simulink model "assignment2_pruned_2022"  (R2022a)
settings: Solver=FixedStepDiscrete  StartTime=0.0  StopTime=1  FixedStep=0.001  RelTol=1e-3
libraries: dspindex x2, my_neural x2, neural x2, simulink x1, dspsigattribs x1, hdlsllib x1, my_support_func x1
settings Model: DataTypeOverride=Off  Creator=13698  LastModifiedBy=omnipresent
settings OptimizationCC: BlockReduction=off  ConditionallyExecuteInputs=off  DefaultParameterBehavior=Inlined  InheritOutputTypeSmallerThanSingle=on
settings DebuggingCC: AlgebraicLoopMsg=error  SingleTaskRateTransMsg=error  ParameterOverflowMsg=none
settings HardwareCC: ProdBitPerPointer=32  ProdBitPerSizeT=32  ProdBitPerPtrDiffT=32  ProdLargestAtomicFloat=None  ProdIntDivRoundTo=Undefined  ProdEndianess=Unspecified  ProdWordSize=32  ProdHWDeviceType=ASIC/FPGA->ASIC/FPGA  TargetBitPerLong=64  TargetBitPerPointer=64  TargetBitPerSizeT=64  TargetBitPerPtrDiffT=64  TargetLongLongMode=on  TargetIntDivRoundTo=Zero  TargetEndianess=LittleEndian  TargetWordSize=64  TargetHWDeviceType=Custom Processor->MATLAB Host Computer  ProdEqTarget=off
settings ModelReferenceCC: EnableRefExpFcnMdlSchedulingChecks=off
settings RTWCC: Description=Generic Real-Time Target

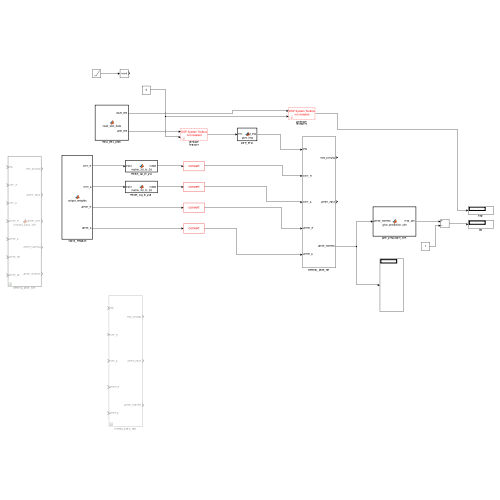
[thumbnail: Simulink's stored preview of the top-level diagram]
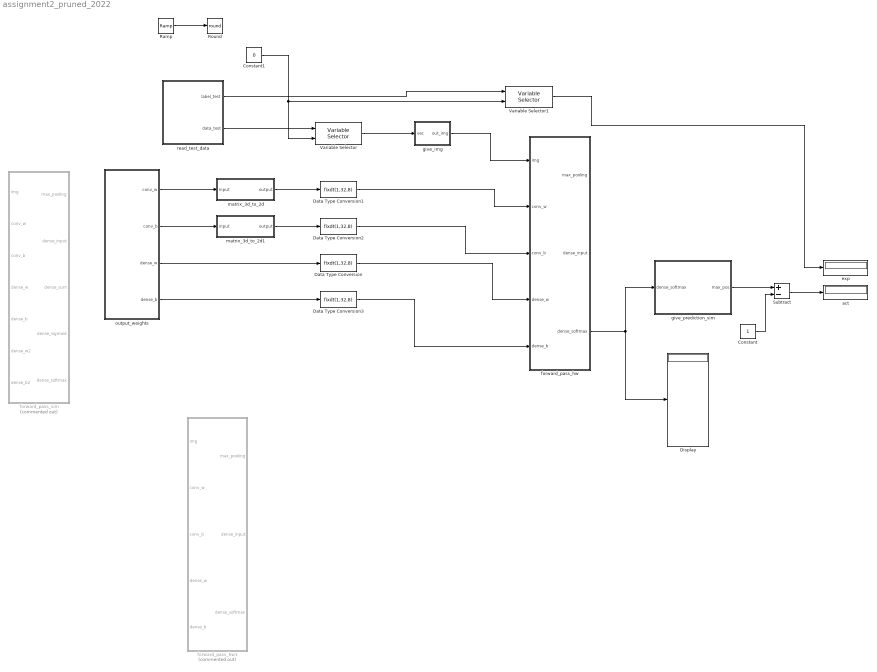
== system assignment2_pruned_2022 ==
  Constant : Constant  OutDataTypeStr=single
  Constant1 : Constant  Value=0
  Data Type Conversion{,1..3} (4 alike) : DataTypeConversion  OutDataTypeStr=fixdt(1,32,8)  SaturateOnIntegerOverflow=off  RndMeth=Floor
  Display : Display
  Ramp : simulink/Sources/Ramp  slope=1  start=0  InitialOutput=0
  Round : Rounding  Operator=round
  Subtract : Sum  Inputs=+-
  Variable Selector : dspindex/Variable Selector  NumInputs=1  rowsOrCols=Rows  IdxMode=Variable  Elements=[1 3]  ZerOneIdxMode=Zero-based  errmode=Generate Error  FillMode=on  FillValues=0
  Variable Selector1 : dspindex/Variable Selector  NumInputs=1  rowsOrCols=Columns  IdxMode=Variable  Elements=[1 3]  ZerOneIdxMode=Zero-based  errmode=Clip Index  FillMode=on  FillValues=0
  act : Display
  exp : Display
  forward_pass_hw : Subsystem
  forward_pass_hw1 : Subsystem  Commented=on
  forward_pass_sim : MATLAB Function  Commented=on  TreatAsAtomicUnit=on
  give_img : MATLAB Function  TreatAsAtomicUnit=on
  give_prediction_sim : MATLAB Function  TreatAsAtomicUnit=on
  matrix_3d_to_2d : MATLAB Function  TreatAsAtomicUnit=on
  matrix_3d_to_2d1 : MATLAB Function  TreatAsAtomicUnit=on
  output_weights : MATLAB Function  TreatAsAtomicUnit=on
  read_test_data : MATLAB Function  TreatAsAtomicUnit=on
  wires:
  Variable Selector/1 -> give_img/1(vec)
  read_test_data/1(label_test) -> Variable Selector1/1
  Variable Selector1/1 -> exp/1
  read_test_data/2(data_test) -> Variable Selector/1
  Subtract/1 -> act/1
  give_prediction_sim/1(max_pos) -> Subtract/1
  Constant/1 -> Subtract/2
  forward_pass_hw/3(dense_softmax) -> Display/1, give_prediction_sim/1(dense_softmax)
  output_weights/3(dense_w) -> Data Type Conversion/1
  output_weights/4(dense_b) -> Data Type Conversion3/1
  Ramp/1 -> Round/1
  Constant1/1 -> Variable Selector1/2, Variable Selector/2
  give_img/1(out_img) -> forward_pass_hw/1(img)
  matrix_3d_to_2d/1(output) -> Data Type Conversion1/1
  matrix_3d_to_2d1/1(output) -> Data Type Conversion2/1
  output_weights/1(conv_w) -> matrix_3d_to_2d/1(input)
  output_weights/2(conv_b) -> matrix_3d_to_2d1/1(input)
  Data Type Conversion/1 -> forward_pass_hw/4(dense_w)
  Data Type Conversion3/1 -> forward_pass_hw/5(dense_b)
  Data Type Conversion1/1 -> forward_pass_hw/2(conv_w)
  Data Type Conversion2/1 -> forward_pass_hw/3(conv_b)

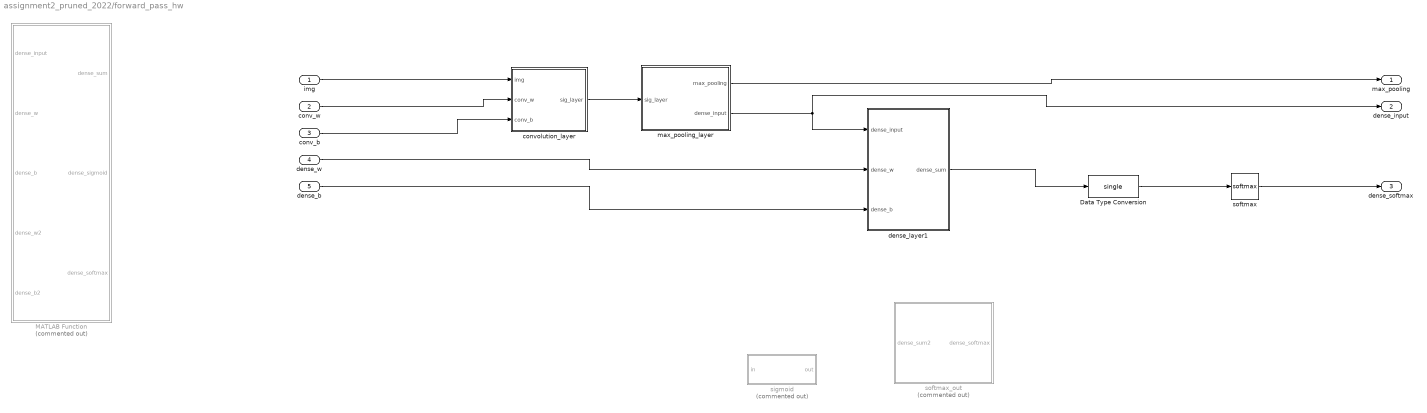
== system assignment2_pruned_2022/forward_pass_hw ==
  img : Inport
  conv_w : Inport  Port=2
  conv_b : Inport  Port=3
  dense_w : Inport  Port=4
  dense_b : Inport  Port=5
  Data Type Conversion : DataTypeConversion  OutDataTypeStr=single  SaturateOnIntegerOverflow=off  RndMeth=Floor
  MATLAB Function : MATLAB Function  Commented=on  TreatAsAtomicUnit=on
  convolution_layer : Subsystem
  dense_layer1 : Subsystem
  max_pooling_layer : MATLAB Function  TreatAsAtomicUnit=on
  sigmoid : Subsystem  Commented=on
  softmax : my_neural/Transfer Functions/softmax
  softmax_out : Subsystem  Commented=on
  max_pooling : Outport
  dense_input : Outport  Port=2
  dense_softmax : Outport  Port=3
  wires:
  convolution_layer/1(sig_layer) -> max_pooling_layer/1(sig_layer)
  max_pooling_layer/2(dense_input) -> dense_layer1/1(dense_input), dense_input/1
  max_pooling_layer/1(max_pooling) -> max_pooling/1
  softmax/1 -> dense_softmax/1
  dense_layer1/1(dense_sum) -> Data Type Conversion/1
  dense_w/1 -> dense_layer1/2(dense_w)
  dense_b/1 -> dense_layer1/3(dense_b)
  conv_w/1 -> convolution_layer/2(conv_w)
  img/1 -> convolution_layer/1(img)
  conv_b/1 -> convolution_layer/3(conv_b)
  Data Type Conversion/1 -> softmax/1

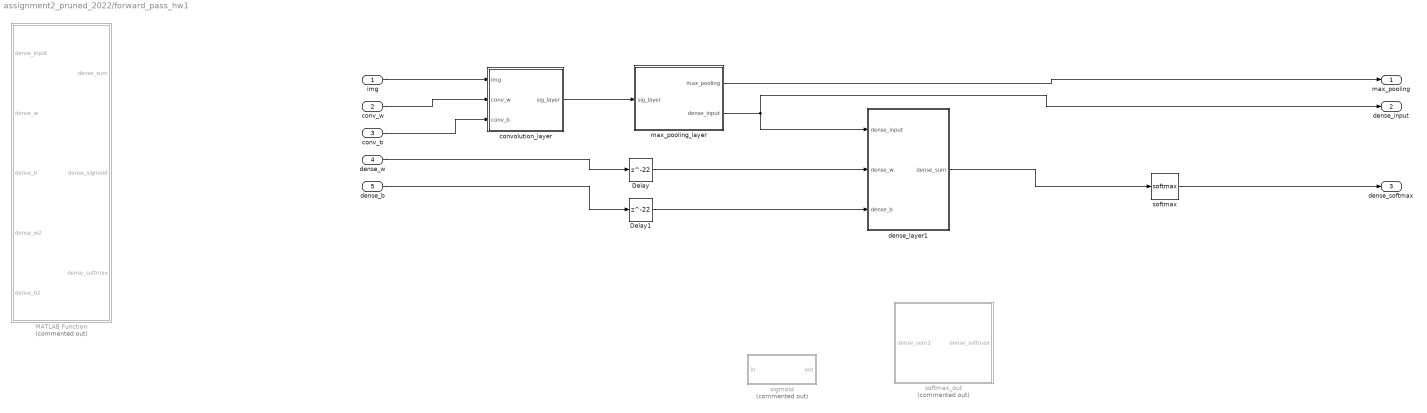
== system assignment2_pruned_2022/forward_pass_hw1 ==
  img : Inport
  conv_w : Inport  Port=2
  conv_b : Inport  Port=3
  dense_w : Inport  Port=4
  dense_b : Inport  Port=5
  Delay : Delay  DelayLength=22
  Delay1 : Delay  DelayLength=22
  MATLAB Function : MATLAB Function  Commented=on  TreatAsAtomicUnit=on
  convolution_layer : Subsystem
  dense_layer1 : Subsystem
  max_pooling_layer : MATLAB Function  TreatAsAtomicUnit=on
  sigmoid : Subsystem  Commented=on
  softmax : neural/Transfer Functions/softmax
  softmax_out : Subsystem  Commented=on
  max_pooling : Outport
  dense_input : Outport  Port=2
  dense_softmax : Outport  Port=3
  wires:
  img/1 -> convolution_layer/1(img)
  conv_w/1 -> convolution_layer/2(conv_w)
  conv_b/1 -> convolution_layer/3(conv_b)
  convolution_layer/1(sig_layer) -> max_pooling_layer/1(sig_layer)
  max_pooling_layer/2(dense_input) -> dense_input/1, dense_layer1/1(dense_input)
  max_pooling_layer/1(max_pooling) -> max_pooling/1
  dense_w/1 -> Delay/1
  dense_b/1 -> Delay1/1
  softmax/1 -> dense_softmax/1
  dense_layer1/1(dense_sum) -> softmax/1
  Delay/1 -> dense_layer1/2(dense_w)
  Delay1/1 -> dense_layer1/3(dense_b)

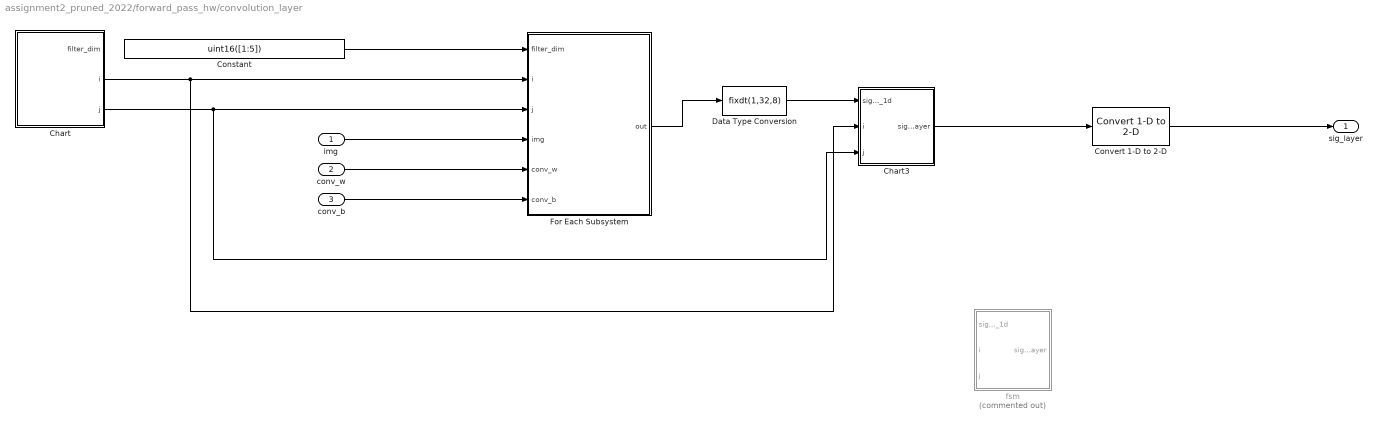
== system assignment2_pruned_2022/forward_pass_hw/convolution_layer ==
  img : Inport
  conv_w : Inport  Port=2
  conv_b : Inport  Port=3
  Chart : Stateflow chart  TreatAsAtomicUnit=on
  Chart3 : Stateflow chart  TreatAsAtomicUnit=on
  Constant : Constant  Value=uint16([1:5])  SampleTime=-1
  Convert 1-D to 2-D : dspsigattribs/Convert 1-D to 2-D  M=5  N=784  frameBasedOut=off
  Data Type Conversion : DataTypeConversion  OutDataTypeStr=fixdt(1,32,8)  SaturateOnIntegerOverflow=off  RndMeth=Floor
  For Each Subsystem : Subsystem  TreatAsAtomicUnit=on
  fsm : Stateflow chart  Commented=on  TreatAsAtomicUnit=on
  sig_layer : Outport
  wires:
  img/1 -> For Each Subsystem/4(img)
  conv_w/1 -> For Each Subsystem/5(conv_w)
  conv_b/1 -> For Each Subsystem/6(conv_b)
  For Each Subsystem/1(out) -> Data Type Conversion/1
  Data Type Conversion/1 -> Chart3/1(sig_layer_1d)
  Chart3/1(sig_layer) -> Convert 1-D to 2-D/1
  Convert 1-D to 2-D/1 -> sig_layer/1
  Chart/3(j) -> Chart3/3(j), For Each Subsystem/3(j)
  Chart/2(i) -> Chart3/2(i), For Each Subsystem/2(i)
  Constant/1 -> For Each Subsystem/1(filter_dim)

== system assignment2_pruned_2022/forward_pass_hw/dense_layer1 ==
  dense_input : Inport
  dense_w : Inport  Port=2
  dense_b : Inport  Port=3
  For Each Subsystem : Subsystem  TreatAsAtomicUnit=on
  dense_sum : Outport
  wires:
  dense_input/1 -> For Each Subsystem/1(dense_input)
  dense_w/1 -> For Each Subsystem/2(dense_w)
  dense_b/1 -> For Each Subsystem/3(dense_b)
  For Each Subsystem/1(dense_sum) -> dense_sum/1

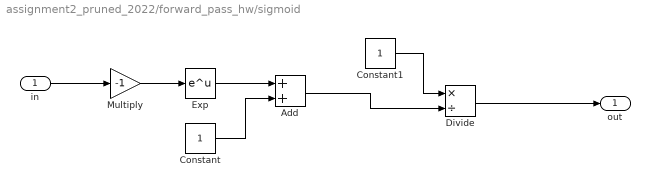
== system assignment2_pruned_2022/forward_pass_hw/sigmoid ==
  in : Inport
  Add : Sum
  Constant : Constant
  Constant1 : Constant
  Divide : Product  Inputs=*/
  Exp : Math
  Multiply : Gain  Gain=-1
  out : Outport
  wires:
  in/1 -> Multiply/1
  Multiply/1 -> Exp/1
  Exp/1 -> Add/1
  Constant/1 -> Add/2
  Divide/1 -> out/1
  Add/1 -> Divide/2
  Constant1/1 -> Divide/1

== system assignment2_pruned_2022/forward_pass_hw/softmax_out ==
  dense_sum2 : Inport
  Exp : Math
  For Each Subsystem : Subsystem  TreatAsAtomicUnit=on
  Sum of Elements : Sum  Inputs=+
  dense_softmax : Outport
  wires:
  dense_sum2/1 -> Exp/1
  Exp/1 -> For Each Subsystem/2(exp_dense_sum2), Sum of Elements/1
  For Each Subsystem/1(dense_softmax) -> dense_softmax/1
  Sum of Elements/1 -> For Each Subsystem/1(den)

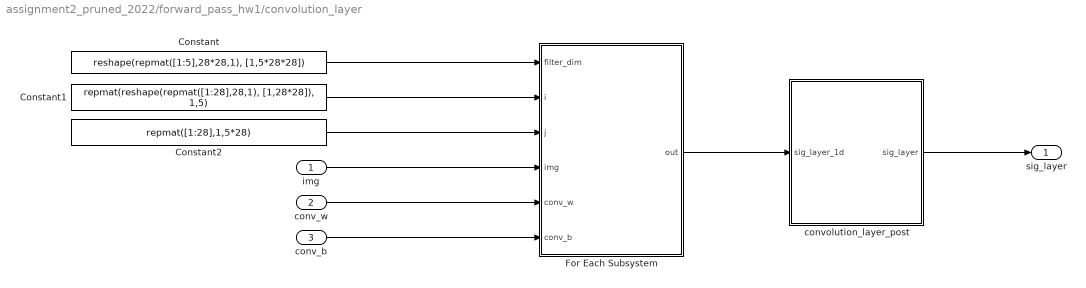
== system assignment2_pruned_2022/forward_pass_hw1/convolution_layer ==
  img : Inport
  conv_w : Inport  Port=2
  conv_b : Inport  Port=3
  Constant : Constant  Value=reshape(repmat([1:5],28*28,1), [1,5*28*28])  OutDataTypeStr=single  SampleTime=-1
  Constant1 : Constant  Value=repmat(reshape(repmat([1:28],28,1), [1,28*28]), 1,5)  OutDataTypeStr=single  SampleTime=-1
  Constant2 : Constant  Value=repmat([1:28],1,5*28)  OutDataTypeStr=single  SampleTime=-1
  For Each Subsystem : Subsystem  TreatAsAtomicUnit=on
  convolution_layer_post : MATLAB Function  TreatAsAtomicUnit=on
  sig_layer : Outport
  wires:
  img/1 -> For Each Subsystem/4(img)
  conv_w/1 -> For Each Subsystem/5(conv_w)
  conv_b/1 -> For Each Subsystem/6(conv_b)
  Constant/1 -> For Each Subsystem/1(filter_dim)
  Constant1/1 -> For Each Subsystem/2(i)
  Constant2/1 -> For Each Subsystem/3(j)
  For Each Subsystem/1(out) -> convolution_layer_post/1(sig_layer_1d)
  convolution_layer_post/1(sig_layer) -> sig_layer/1

== system assignment2_pruned_2022/forward_pass_hw1/dense_layer1 ==
  dense_input : Inport
  dense_w : Inport  Port=2
  dense_b : Inport  Port=3
  For Each Subsystem : Subsystem  TreatAsAtomicUnit=on
  dense_sum : Outport
  wires:
  dense_input/1 -> For Each Subsystem/1(dense_input)
  dense_w/1 -> For Each Subsystem/2(dense_w)
  dense_b/1 -> For Each Subsystem/3(dense_b)
  For Each Subsystem/1(dense_sum) -> dense_sum/1

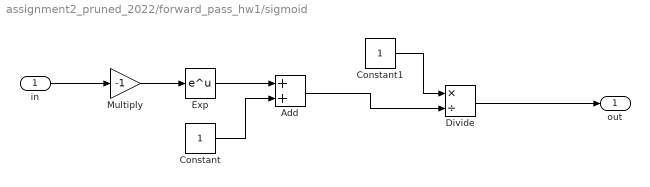
== system assignment2_pruned_2022/forward_pass_hw1/sigmoid ==
  in : Inport
  Add : Sum
  Constant : Constant
  Constant1 : Constant
  Divide : Product  Inputs=*/
  Exp : Math
  Multiply : Gain  Gain=-1
  out : Outport
  wires:
  in/1 -> Multiply/1
  Multiply/1 -> Exp/1
  Exp/1 -> Add/1
  Constant/1 -> Add/2
  Divide/1 -> out/1
  Add/1 -> Divide/2
  Constant1/1 -> Divide/1

== system assignment2_pruned_2022/forward_pass_hw1/softmax_out ==
  dense_sum2 : Inport
  Exp : Math
  For Each Subsystem : Subsystem  TreatAsAtomicUnit=on
  Sum of Elements : Sum  Inputs=+
  dense_softmax : Outport
  wires:
  dense_sum2/1 -> Exp/1
  Exp/1 -> For Each Subsystem/2(exp_dense_sum2), Sum of Elements/1
  For Each Subsystem/1(dense_softmax) -> dense_softmax/1
  Sum of Elements/1 -> For Each Subsystem/1(den)

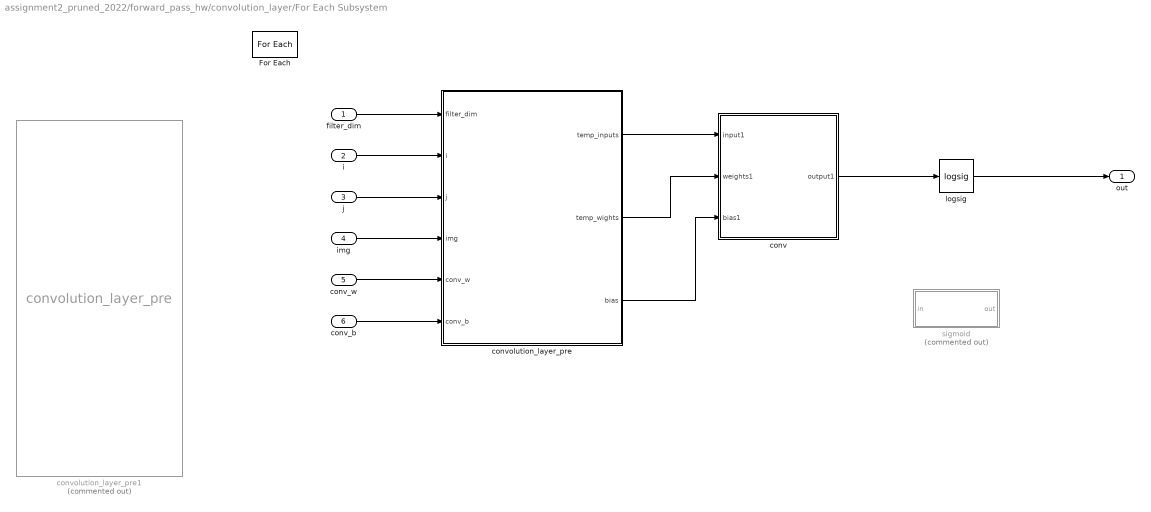
== system assignment2_pruned_2022/forward_pass_hw/convolution_layer/For Each Subsystem ==
  filter_dim : Inport  Partition=on  PartitionDimension=1  PartitionWidth=1  PartitionOffset=0
  i : Inport  Port=2
  j : Inport  Port=3
  img : Inport  Port=4
  conv_w : Inport  Port=5
  conv_b : Inport  Port=6
  For Each : ForEach  DisableCoverage=on
  conv : Subsystem
  convolution_layer_pre : MATLAB Function  TreatAsAtomicUnit=on
  convolution_layer_pre1 : my_support_func/convolution_layer_pre  Commented=on  SampleTime=-1
  logsig : my_neural/Transfer Functions/logsig
  sigmoid : Subsystem  Commented=on
  out : Outport  ConcatenationDimension=1
  wires:
  logsig/1 -> out/1
  conv/1(output1) -> logsig/1
  filter_dim/1 -> convolution_layer_pre/1(filter_dim)
  i/1 -> convolution_layer_pre/2(i)
  j/1 -> convolution_layer_pre/3(j)
  img/1 -> convolution_layer_pre/4(img)
  conv_w/1 -> convolution_layer_pre/5(conv_w)
  conv_b/1 -> convolution_layer_pre/6(conv_b)
  convolution_layer_pre/1(temp_inputs) -> conv/1(input1)
  convolution_layer_pre/2(temp_wights) -> conv/2(weights1)
  convolution_layer_pre/3(bias) -> conv/3(bias1)

== system assignment2_pruned_2022/forward_pass_hw/dense_layer1/For Each Subsystem ==
  dense_input : Inport
  dense_w : Inport  Port=2  Partition=on  PartitionDimension=2  PartitionWidth=1  PartitionOffset=0
  dense_b : Inport  Port=3  Partition=on  PartitionDimension=2  PartitionWidth=1  PartitionOffset=0
  For Each : ForEach  DisableCoverage=on
  conv : Subsystem
  dense_sum : Outport  ConcatenationDimension=1
  wires:
  dense_input/1 -> conv/1(input)
  dense_b/1 -> conv/3(bias)
  conv/1(output) -> dense_sum/1
  dense_w/1 -> conv/2(weights)

== system assignment2_pruned_2022/forward_pass_hw/softmax_out/For Each Subsystem ==
  den : Inport
  exp_dense_sum2 : Inport  Port=2  Partition=on  PartitionDimension=1  PartitionWidth=1  PartitionOffset=0
  Divide : Product  Inputs=*/
  For Each : ForEach  DisableCoverage=on
  dense_softmax : Outport  ConcatenationDimension=1
  wires:
  Divide/1 -> dense_softmax/1
  exp_dense_sum2/1 -> Divide/1
  den/1 -> Divide/2

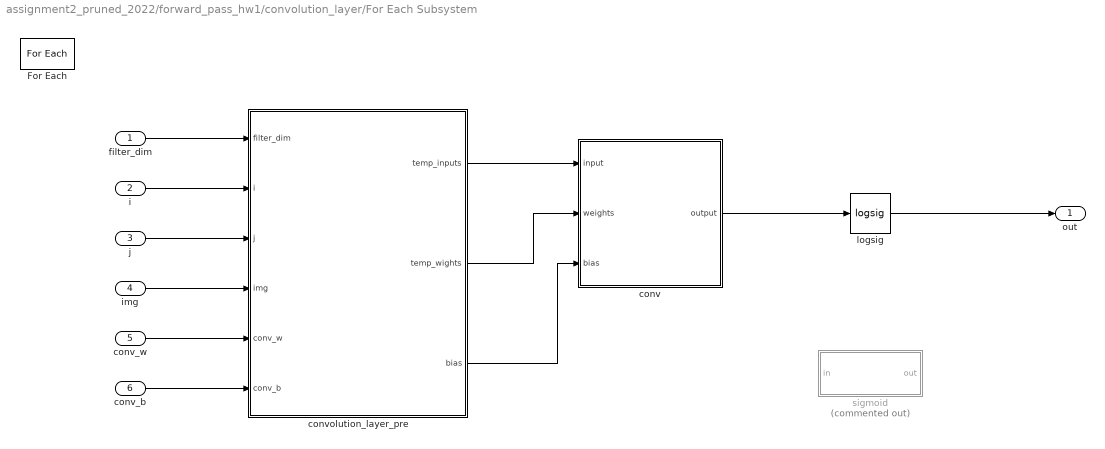
== system assignment2_pruned_2022/forward_pass_hw1/convolution_layer/For Each Subsystem ==
  filter_dim : Inport  Partition=on  PartitionDimension=1  PartitionWidth=1  PartitionOffset=0
  i : Inport  Port=2  Partition=on  PartitionDimension=1  PartitionWidth=1  PartitionOffset=0
  j : Inport  Port=3  Partition=on  PartitionDimension=1  PartitionWidth=1  PartitionOffset=0
  img : Inport  Port=4
  conv_w : Inport  Port=5
  conv_b : Inport  Port=6
  For Each : ForEach  DisableCoverage=on
  conv : Subsystem
  convolution_layer_pre : MATLAB Function  TreatAsAtomicUnit=on
  logsig : neural/Transfer Functions/logsig
  sigmoid : Subsystem  Commented=on
  out : Outport  ConcatenationDimension=1
  wires:
  convolution_layer_pre/1(temp_inputs) -> conv/1(input)
  convolution_layer_pre/2(temp_wights) -> conv/2(weights)
  convolution_layer_pre/3(bias) -> conv/3(bias)
  filter_dim/1 -> convolution_layer_pre/1(filter_dim)
  i/1 -> convolution_layer_pre/2(i)
  j/1 -> convolution_layer_pre/3(j)
  img/1 -> convolution_layer_pre/4(img)
  conv_w/1 -> convolution_layer_pre/5(conv_w)
  conv_b/1 -> convolution_layer_pre/6(conv_b)
  conv/1(output) -> logsig/1
  logsig/1 -> out/1

== system assignment2_pruned_2022/forward_pass_hw1/dense_layer1/For Each Subsystem ==
  dense_input : Inport
  dense_w : Inport  Port=2  Partition=on  PartitionDimension=2  PartitionWidth=1  PartitionOffset=0
  dense_b : Inport  Port=3  Partition=on  PartitionDimension=2  PartitionWidth=1  PartitionOffset=0
  For Each : ForEach  DisableCoverage=on
  conv : Subsystem
  dense_sum : Outport  ConcatenationDimension=1
  wires:
  dense_input/1 -> conv/1(input)
  dense_b/1 -> conv/3(bias)
  conv/1(output) -> dense_sum/1
  dense_w/1 -> conv/2(weights)

== system assignment2_pruned_2022/forward_pass_hw1/softmax_out/For Each Subsystem ==
  den : Inport
  exp_dense_sum2 : Inport  Port=2  Partition=on  PartitionDimension=1  PartitionWidth=1  PartitionOffset=0
  Divide : Product  Inputs=*/
  For Each : ForEach  DisableCoverage=on
  dense_softmax : Outport  ConcatenationDimension=1
  wires:
  Divide/1 -> dense_softmax/1
  exp_dense_sum2/1 -> Divide/1
  den/1 -> Divide/2

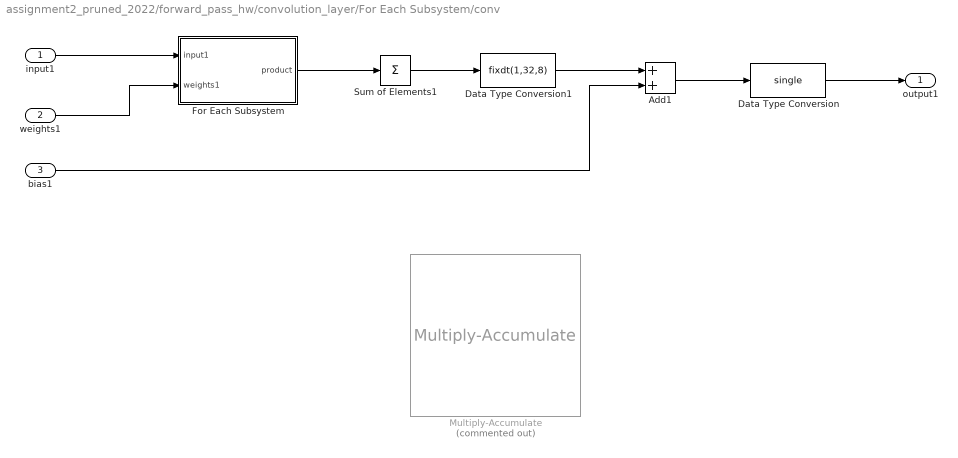
== system assignment2_pruned_2022/forward_pass_hw/convolution_layer/For Each Subsystem/conv ==
  input1 : Inport
  weights1 : Inport  Port=2
  bias1 : Inport  Port=3
  Add1 : Sum
  Data Type Conversion : DataTypeConversion  OutDataTypeStr=single  SaturateOnIntegerOverflow=off  RndMeth=Floor
  Data Type Conversion1 : DataTypeConversion  OutDataTypeStr=fixdt(1,32,8)  SaturateOnIntegerOverflow=off  RndMeth=Floor
  For Each Subsystem : Subsystem  TreatAsAtomicUnit=on
  Multiply-Accumulate : hdlsllib/HDL Operations/Multiply-Accumulate  Commented=on  opMode=Vector  initValueSetting=Input port  initValue=0  initValueSetting2=Dialog  initValue2=0  initValueSetting3=Dialog  initValue3=0  num_samples=2  RndMeth2=Floor  RndMeth3=Floor  OutDataTypeStr=fixdt(1,32,8)  datatype2=Inherit: Inherit via back propagation  datatype3=Inherit: Inherit via back propagation  validOut=on  endInandOut=on  startOut=on  countOut=on  dim=-1  DoSatur=off  parallel=off
  Sum of Elements1 : Sum  Inputs=+
  output1 : Outport
  wires:
  Sum of Elements1/1 -> Data Type Conversion1/1
  bias1/1 -> Add1/2
  Add1/1 -> Data Type Conversion/1
  input1/1 -> For Each Subsystem/1(input1)
  weights1/1 -> For Each Subsystem/2(weights1)
  For Each Subsystem/1(product) -> Sum of Elements1/1
  Data Type Conversion/1 -> output1/1
  Data Type Conversion1/1 -> Add1/1

== system assignment2_pruned_2022/forward_pass_hw/convolution_layer/For Each Subsystem/sigmoid ==
  in : Inport
  Add : Sum
  Constant : Constant
  Constant1 : Constant
  Divide : Product  Inputs=*/
  Exp : Math
  Multiply : Gain  Gain=-1
  out : Outport
  wires:
  in/1 -> Multiply/1
  Multiply/1 -> Exp/1
  Exp/1 -> Add/1
  Constant/1 -> Add/2
  Divide/1 -> out/1
  Add/1 -> Divide/2
  Constant1/1 -> Divide/1

== system assignment2_pruned_2022/forward_pass_hw/dense_layer1/For Each Subsystem/conv ==
  input : Inport
  weights : Inport  Port=2
  bias : Inport  Port=3
  Add : Sum  OutDataTypeStr=Inherit: Inherit via back propagation
  Data Type Conversion : DataTypeConversion  OutDataTypeStr=fixdt(1,32,8)  SaturateOnIntegerOverflow=off  RndMeth=Floor
  For Each Subsystem : Subsystem  TreatAsAtomicUnit=on
  Sum of Elements : Sum  Inputs=+
  output : Outport
  wires:
  Add/1 -> output/1
  Sum of Elements/1 -> Data Type Conversion/1
  bias/1 -> Add/2
  For Each Subsystem/1(product) -> Sum of Elements/1
  input/1 -> For Each Subsystem/1(input1)
  weights/1 -> For Each Subsystem/2(weights1)
  Data Type Conversion/1 -> Add/1

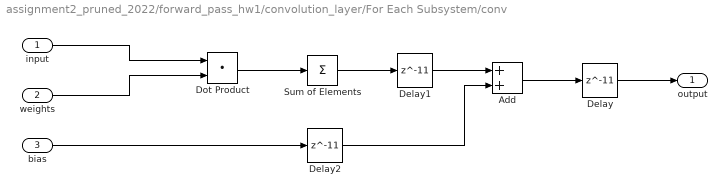
== system assignment2_pruned_2022/forward_pass_hw1/convolution_layer/For Each Subsystem/conv ==
  input : Inport
  weights : Inport  Port=2
  bias : Inport  Port=3
  Add : Sum
  Delay : Delay  DelayLength=11
  Delay1 : Delay  DelayLength=11
  Delay2 : Delay  DelayLength=11
  Dot Product : DotProduct  OutDataTypeStr=Inherit: Inherit via internal rule
  Sum of Elements : Sum  Inputs=+
  output : Outport
  wires:
  input/1 -> Dot Product/1
  weights/1 -> Dot Product/2
  Dot Product/1 -> Sum of Elements/1
  Sum of Elements/1 -> Delay1/1
  bias/1 -> Delay2/1
  Delay/1 -> output/1
  Delay1/1 -> Add/1
  Delay2/1 -> Add/2
  Add/1 -> Delay/1

== system assignment2_pruned_2022/forward_pass_hw1/convolution_layer/For Each Subsystem/sigmoid ==
  in : Inport
  Add : Sum
  Constant : Constant
  Constant1 : Constant
  Divide : Product  Inputs=*/
  Exp : Math
  Multiply : Gain  Gain=-1
  out : Outport
  wires:
  in/1 -> Multiply/1
  Multiply/1 -> Exp/1
  Exp/1 -> Add/1
  Constant/1 -> Add/2
  Divide/1 -> out/1
  Add/1 -> Divide/2
  Constant1/1 -> Divide/1

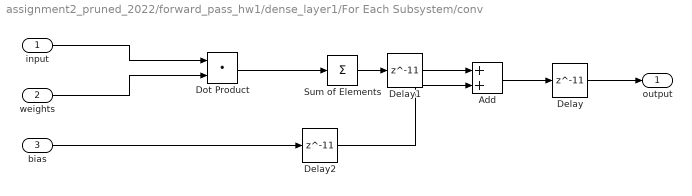
== system assignment2_pruned_2022/forward_pass_hw1/dense_layer1/For Each Subsystem/conv ==
  input : Inport
  weights : Inport  Port=2
  bias : Inport  Port=3
  Add : Sum  OutDataTypeStr=single
  Delay : Delay  DelayLength=11
  Delay1 : Delay  DelayLength=11
  Delay2 : Delay  DelayLength=11
  Dot Product : DotProduct  OutDataTypeStr=Inherit: Inherit via internal rule
  Sum of Elements : Sum  Inputs=+
  output : Outport
  wires:
  input/1 -> Dot Product/1
  weights/1 -> Dot Product/2
  Dot Product/1 -> Sum of Elements/1
  Sum of Elements/1 -> Delay1/1
  Add/1 -> Delay/1
  bias/1 -> Delay2/1
  Delay/1 -> output/1
  Delay1/1 -> Add/1
  Delay2/1 -> Add/2

== system assignment2_pruned_2022/forward_pass_hw/convolution_layer/For Each Subsystem/conv/For Each Subsystem ==
  input1 : Inport  Partition=on  PartitionDimension=2  PartitionWidth=1  PartitionOffset=0
  weights1 : Inport  Port=2  Partition=on  PartitionDimension=2  PartitionWidth=1  PartitionOffset=0
  For Each : ForEach  DisableCoverage=on
  Product : Product
  product : Outport  ConcatenationDimension=1
  wires:
  input1/1 -> Product/1
  weights1/1 -> Product/2
  Product/1 -> product/1

== system assignment2_pruned_2022/forward_pass_hw/dense_layer1/For Each Subsystem/conv/For Each Subsystem ==
  input1 : Inport  Partition=on  PartitionDimension=2  PartitionWidth=1  PartitionOffset=0
  weights1 : Inport  Port=2  Partition=on  PartitionDimension=1  PartitionWidth=1  PartitionOffset=0
  For Each : ForEach  DisableCoverage=on
  Product : Product
  product : Outport  ConcatenationDimension=1
  wires:
  input1/1 -> Product/1
  weights1/1 -> Product/2
  Product/1 -> product/1

== matlab function assignment2_pruned_2022/read_test_data ==
  data: label_test output; data_test output
function [label_test, data_test] = read_test_data()
    data = load('test_set.mat');
    label_test = data.label_test;
    data_test = data.data_test;
end

== matlab function assignment2_pruned_2022/output_weights ==
  data: conv_w output; conv_b output; dense_w output; dense_b output
function [conv_w, conv_b, dense_w, dense_b] = output_weights
    data = load('weights_pruned.mat');
    conv_w = (data.conv_w);
    conv_b = (data.conv_b);
    dense_w = (data.dense_w);
    dense_b = (data.dense_b);
    end

== matlab function assignment2_pruned_2022/give_img ==
  data: vec input; out_img output
function out_img = give_img(vec)
    img = zeros(35,32,'uint8');
    k=1;
    for i=1:35
        for j=1:32
            if (i < 6|| j < 3 || i > 33 || j > 30)
                img(i,j) = 0;
            else
                img(i,j) = vec(k);
                k = k + 1;
            end
        end
    end

    out_img = reshape(transpose(img), [1, length(img(1,:))*length(img)]);
end

== matlab function assignment2_pruned_2022/forward_pass_hw/convolution_layer/For Each Subsystem/convolution_layer_pre ==
  settings: fimath=fimath('RoundingMethod', 'Floor','OverflowAction', 'Wrap','ProductMode', 'FullPrecision', 'SumMode', 'FullPrecision')
  data: filter_dim input; temp_inputs output; i input; j input; img input; conv_w input; conv_b input; temp_wights output; bias output
function [temp_inputs, temp_wights, bias] = convolution_layer_pre(filter_dim, i, j, img, conv_w, conv_b)
    
    % temp_img = reshape(transpose(img), [1, length(img(1,:))*length(img)]);
    
    temp_wights = fi(zeros(1,7*7), 1, 32, 8);
    temp_inputs = fi(zeros(1,7*7), 1, 32, 8);
    i = single(i);
    j = single(j);
    for k=1:7
        for l=1:7
            temp_wights((k-1)*7 + l) = single(img((i + k + 1 - 1 - 1)*32 + j + l - 2 - 1));
            temp_inputs((k-1)*7 + l) = conv_w(filter_dim, (k-1)*7 + l);
        end
    end
    bias = conv_b(filter_dim, (i-1)*28+j);
    
    % temp_wights = zeros(1,7*7, "single");
    % temp_inputs = zeros(1,7*7, "single");
    % for k=1:7
    %     for l=1:7
    %         temp_wights((k-1)*7 + l) = cast(img((i + k + 1 - 1 - 1)*32 + j + l - 2 - 1), 'double');
    %         temp_inputs((k-1)*7 + l) = conv_w(filter_dim, k, l);
    %     end
    % end
    % bias = conv_b(filter_dim, i, j);
end

== matlab function assignment2_pruned_2022/forward_pass_sim ==
  data: img input; max_pooling output; conv_w input; conv_b input; dense_w input; dense_b input; dense_w2 input; dense_b2 input; dense_input output; dense_sum output; dense_sigmoid output; dense_softmax output
function [max_pooling, dense_input, dense_sum, dense_sigmoid, dense_softmax] = forward_pass_sim(img, conv_w, conv_b, dense_w, dense_b, dense_w2, dense_b2)
    max_pooling = zeros(5,28,28);
    dense_input = zeros(1,980);
    dense_sum = zeros(1,120);
    dense_sigmoid = zeros(1,120);
    dense_softmax = zeros(1,10);
    
    conv_layer = zeros(5,28,28);
    sig_layer = zeros(5,28,28);
    max_layer = zeros(5,14,14);
    dense_sum2 = zeros(1,10);
    
    temp_img = reshape(transpose(img), [1, length(img(1,:))*length(img)]);
    
    % Convolution Operation + Sigmoid Activation
    for filter_dim=1:5
        for i=1:28
            for j=1:28
                temp_wights = zeros(1,7*7);
                temp_inputs = zeros(1,7*7);
                for k=1:7
                    for l=1:7
                        temp_wights((k-1)*7 + l) = cast(temp_img((i + k + 1 - 1 - 1)*32 + j + l - 2 - 1), 'double');
                        temp_inputs((k-1)*7 + l) = conv_w(filter_dim, k, l);
                    end
                end
                conv_layer(filter_dim, i, j) = convolusion(temp_inputs, temp_wights, conv_b(filter_dim, i, j));
            end
        end
    end
    sig_layer = 1 ./ (1 + exp(-1 .* conv_layer));
    
    % MAX Pooling (max_pooling, max_layer)
    for filter_dim=1:5
        for i=1:2:28
            for j=1:2:28
                matrix = sig_layer(filter_dim,i:i+1,j:j+1);
                [M,I] = max(matrix);
                [M2,I2] = max(M);
                I = [I(I2) I2];
                max_pooling(filter_dim, I(1), I(2)) = 1;
                max_layer(filter_dim, (i+1)/2, (j+1)/2) = M2;
            end
        end
    end
    for i=1:5
        for j=1:14
            dense_input((i-1)*14*14 + (j-1)*14 + 1 : (i-1)*14*14 + (j-1)*14 + 14) = reshape(max_layer(i,j,:), [1 14]);
        end
    end
    
    % Dense Layer
    for i=1:120
        dense_sum(i) = convolusion(transpose(dense_w(:,i)), dense_input, dense_b(i));
    end
    dense_sigmoid = 1 ./ (1 + exp(-1 .* dense_sum));
    
    % Dense Layer 2
    for i=1:10
        dense_sum2(i) = convolusion(transpose(dense_w2(:,i)), dense_sigmoid, dense_b2(i));
    end
    
    % Softmax Output
    dense_softmax_new = exp(dense_sum2);
    for i=1:10
        dense_softmax(i) = dense_softmax_new(i) / sum(dense_softmax_new);
    end
end

== matlab function assignment2_pruned_2022/forward_pass_hw/MATLAB Function ==
  settings: fimath=fimath('RoundingMethod', 'Floor','OverflowAction', 'Wrap','ProductMode', 'FullPrecision', 'SumMode', 'FullPrecision')
  data: dense_input input; dense_w input; dense_b input; dense_w2 input; dense_b2 input; dense_sum output; dense_sigmoid output; dense_softmax output
function [dense_sum, dense_sigmoid, dense_softmax] = temp(dense_input, dense_w, dense_b, dense_w2, dense_b2)
max_pooling = zeros(5,28,28);
dense_sum = zeros(1,120);
dense_sigmoid = zeros(1,120);
dense_softmax = zeros(1,10);

conv_layer = zeros(5,28,28);
max_layer = zeros(5,14,14);
dense_sum2 = zeros(1,10);

% Dense Layer
for i=1:120
    dense_sum(i) = convolusion(transpose(dense_w(:,i)), dense_input, dense_b(i));
end
dense_sigmoid = 1 ./ (1 + exp(-1 .* dense_sum));

% Dense Layer 2
for i=1:10
    dense_sum2(i) = convolusion(transpose(dense_w2(:,i)), dense_sigmoid, dense_b2(i));
end

% Softmax Output
dense_softmax_new = exp(dense_sum2);
for i=1:10
    dense_softmax(i) = dense_softmax_new(i) / sum(dense_softmax_new);
end

== matlab function assignment2_pruned_2022/forward_pass_hw/max_pooling_layer ==
  settings: fimath=fimath('RoundingMethod', 'Floor','OverflowAction', 'Wrap','ProductMode', 'FullPrecision', 'SumMode', 'FullPrecision')
  data: sig_layer input; max_pooling output; dense_input output
function [max_pooling, dense_input] = max_pooling_layer(sig_layer)

    max_pooling = fi(zeros(5,28*28), 1, 32, 8);
    max_layer = fi(zeros(5,14*14), 1, 32, 8);
    dense_input = fi(zeros(1,980), 1, 32, 8);
    
    % MAX Pooling (max_pooling, max_layer)
    for filter_dim=uint32(1:5)
        for i=uint32(1:2:28)
            for j=uint32(1:2:28)
                matrix = [sig_layer(filter_dim, (i-1)*28+j), sig_layer(filter_dim, (i-1)*28+j+1), sig_layer(filter_dim, (i)*28+j), sig_layer(filter_dim, (i)*28+j+1)];
                M = max(matrix);
                if (M == matrix(1))
                    I = single(1);
                elseif (M == matrix(2))
                    I = single(2);
                elseif (M == matrix(3))
                    I = single(3);
                else
                    I = single(4);
                end
                max_i = uint32(single(i) + ceil(I/2) - 1);
                max_j = uint32(single(j) + 2-mod(I,2) - 1);
                max_pooling(filter_dim, (max_i-1)*28+max_j) = 1;
                max_layer(filter_dim, ((i+1)/2-1)*14+(j+1)/2) = M;
            end
        end
    end
    for i=uint32(1:5)
        dense_input((i-1)*14*14 + 1 : (i-1)*14*14 + 14*14) = reshape(max_layer(i,:), [1 14*14]);
    end
    
    % pooling = zeros(5,28,28, "single");
    % max_layer = zeros(5,14,14, "single");
    % dense_input = zeros(1,980, "single");
    % 
    % % MAX Pooling (max_pooling, max_layer)
    % for filter_dim=1:5
    %     for i=1:2:28
    %         for j=1:2:28
    %             matrix = sig_layer(filter_dim,i:i+1,j:j+1);
    %             [M,I] = max(matrix);
    %             [M2,I2] = max(M);
    %             I = [I(I2) I2];
    %             max_pooling(filter_dim, I(1), I(2)) = 1;
    %             max_layer(filter_dim, (i+1)/2, (j+1)/2) = M2;
    %         end
    %     end
    % end
    % for i=1:5
    %     for j=1:14
    %         dense_input((i-1)*14*14 + (j-1)*14 + 1 : (i-1)*14*14 + (j-1)*14 + 14) = reshape(max_layer(i,j,:), [1 14]);
    %     end
    % end
end

== matlab function assignment2_pruned_2022/give_prediction_sim ==
  data: dense_softmax input; max_pos output
function max_pos = give_prediction_sim(dense_softmax)
    [~,max_pos] = max(dense_softmax);
end

== matlab function assignment2_pruned_2022/matrix_3d_to_2d ==
  data: input input; output output
function output = matrix_3d_to_2d(input)
    matrix_size = size(input);
    output = zeros([matrix_size(1), matrix_size(2) * matrix_size(3)], 'single');
    for i=1:matrix_size(1)
        for j=1:matrix_size(2)
            output(i, (j-1)*matrix_size(3) + 1 : (j)*matrix_size(3) ) = input(i,j,:);
        end
    end
end

== matlab function assignment2_pruned_2022/matrix_3d_to_2d1 ==
  data: input input; output output
function output = matrix_3d_to_2d(input)
    matrix_size = size(input);
    output = zeros([matrix_size(1), matrix_size(2) * matrix_size(3)], 'single');
    for i=1:matrix_size(1)
        for j=1:matrix_size(2)
            output(i, (j-1)*matrix_size(3) + 1 : (j)*matrix_size(3) ) = input(i,j,:);
        end
    end
end

== stateflow chart assignment2_pruned_2022/forward_pass_hw/convolution_layer/Chart ==
  settings: executeAtInitialization=1
  state init
    filter_dim = 1;
    i = 1;
    j = 1;
  state temp
    i=1;
    j=1;
  state temp1
    i=1;
    j=1;
  state jIncrease
    if (j < 28)
    j = j + 1;
    else
    j = 1;
    end
  state done
  state iIncrease
    if (i < 28)
    i = i + 1;
    else
    i = 1;
    end
  (default) -> init
  init -> temp
  temp -> temp1
  temp1 -> jIncrease
  jIncrease -> jIncrease [order 3]
  jIncrease -> done [order 2] : [i>=28 && j>=28]
  iIncrease -> jIncrease
  jIncrease -> iIncrease [order 1] : [j==1]
  data: filter_dim output uint8; i output uint16; j output uint16

== matlab function assignment2_pruned_2022/forward_pass_hw1/MATLAB Function ==
  settings: fimath=fimath('RoundingMethod', 'Floor','OverflowAction', 'Wrap','ProductMode', 'FullPrecision', 'SumMode', 'FullPrecision')
  data: dense_input input; dense_w input; dense_b input; dense_w2 input; dense_b2 input; dense_sum output; dense_sigmoid output; dense_softmax output
function [dense_sum, dense_sigmoid, dense_softmax] = temp(dense_input, dense_w, dense_b, dense_w2, dense_b2)
max_pooling = zeros(5,28,28);
dense_sum = zeros(1,120);
dense_sigmoid = zeros(1,120);
dense_softmax = zeros(1,10);

conv_layer = zeros(5,28,28);
max_layer = zeros(5,14,14);
dense_sum2 = zeros(1,10);

% Dense Layer
for i=1:120
    dense_sum(i) = convolusion(transpose(dense_w(:,i)), dense_input, dense_b(i));
end
dense_sigmoid = 1 ./ (1 + exp(-1 .* dense_sum));

% Dense Layer 2
for i=1:10
    dense_sum2(i) = convolusion(transpose(dense_w2(:,i)), dense_sigmoid, dense_b2(i));
end

% Softmax Output
dense_softmax_new = exp(dense_sum2);
for i=1:10
    dense_softmax(i) = dense_softmax_new(i) / sum(dense_softmax_new);
end

== stateflow chart assignment2_pruned_2022/forward_pass_hw/convolution_layer/fsm ==
  settings: updateMethod=DISCRETE  executeAtInitialization=1
  state idle
  state update
  state update_value [function]
    (default) -> (junction 536) : {
        |   sig_layer[0][(i-1)*28 + j-1] = sig_layer_1d[0];
        |   sig_layer[1][(i-1)*28 + j-1] = sig_layer_1d[1];
        |   sig_layer[2][(i-1)*28 + j-1] = sig_layer_1d[2];
        |   sig_layer[3][(i-1)*28 + j-1] = sig_layer_1d[3];
        |   sig_layer[4][(i-1)*28 + j-1] = sig_layer_1d[4];
        | }
  state done_update
  state done
  (default) -> idle
  update -> update [order 2] : {update_value();}
  idle -> update : [i != 0 && j != 0]
  update -> done_update [order 1] : [i>=28 && j>=28]{update_value();}
  done_update -> done
  data: sig_layer_1d input fixdt(1,32,8) size=5; i input uint16; j input uint16; sig_layer output fixdt(1,32,8) size=[5 784]

== stateflow chart assignment2_pruned_2022/forward_pass_hw/convolution_layer/Chart3 ==
  settings: executeAtInitialization=1
  state init
  state update
    if (i~=0 && j~=0)
    for filter_dim = uint16(1:5)
    sig_layer((i-1)*28*5 + (j-1)*5 + filter_dim) = sig_layer_1d(filter_dim);
    % fprintf("%u %u %u = %f\n", filter_dim, i, j, sig_layer_1d(filter_dim));
    end
    end
  state done
    if (i~=0 && j~=0)
    for filter_dim = uint16(1:5)
    sig_layer((i-1)*28*5 + (j-1)*5 + filter_dim) = sig_layer_1d(filter_dim);
    % fprintf("%u %u %u = %f\n", filter_dim, i, j, sig_layer_1d(filter_dim));
    end
    end
  state doneIdle
    %fprintf("done conv post\n");
  (default) -> init
  init -> update
  update -> done [order 1] : [i>=28 && j>=28]
  done -> doneIdle
  update -> update [order 2]
  data: sig_layer output fixdt(1,32,8) size=3920; sig_layer_1d input fixdt(1,32,8) size=5; i input uint16; j input uint16; temp local uint16; filter_dim local uint16

== matlab function assignment2_pruned_2022/forward_pass_hw1/convolution_layer/For Each Subsystem/convolution_layer_pre ==
  settings: fimath=fimath('RoundingMethod', 'Floor','OverflowAction', 'Wrap','ProductMode', 'FullPrecision', 'SumMode', 'FullPrecision')
  data: filter_dim input; temp_inputs output; i input; j input; img input; conv_w input; conv_b input; temp_wights output; bias output
function [temp_inputs, temp_wights, bias] = convolution_layer_pre(filter_dim, i, j, img, conv_w, conv_b)

% temp_img = reshape(transpose(img), [1, length(img(1,:))*length(img)]);

temp_wights = zeros(1,7*7, "single");
temp_inputs = zeros(1,7*7, "single");
for k=1:7
    for l=1:7
        temp_wights((k-1)*7 + l) = single(img((i + k + 1 - 1 - 1)*32 + j + l - 2 - 1));
        temp_inputs((k-1)*7 + l) = conv_w(filter_dim, (k-1)*7 + l);
    end
end
bias = conv_b(filter_dim, (i-1)*28+j);

% temp_wights = zeros(1,7*7, "single");
% temp_inputs = zeros(1,7*7, "single");
% for k=1:7
%     for l=1:7
%         temp_wights((k-1)*7 + l) = cast(img((i + k + 1 - 1 - 1)*32 + j + l - 2 - 1), 'double');
%         temp_inputs((k-1)*7 + l) = conv_w(filter_dim, k, l);
%     end
% end
% bias = conv_b(filter_dim, i, j);

== matlab function assignment2_pruned_2022/forward_pass_hw1/convolution_layer/convolution_layer_post ==
  settings: fimath=fimath('RoundingMethod', 'Floor','OverflowAction', 'Wrap','ProductMode', 'FullPrecision', 'SumMode', 'FullPrecision')
  data: sig_layer_1d input; sig_layer output
function sig_layer = convolution_layer_post(sig_layer_1d)

sig_layer = zeros(5,28*28, "single");
for filter_dim=1:5
    sig_layer(filter_dim, :) = sig_layer_1d((filter_dim-1)*28*28 + 1 : (filter_dim-1)*28*28 + 28*28);
end

% sig_layer = zeros(5,28,28, "single");
% for filter_dim=1:5
%     for i=1:28
%         sig_layer(filter_dim, i, :) = sig_layer_1d((filter_dim-1)*28*28 + (i-1)*28 + 1 : (filter_dim-1)*28*28 + (i-1)*28 + 28);
%     end
% end

== matlab function assignment2_pruned_2022/forward_pass_hw1/max_pooling_layer ==
  settings: fimath=fimath('RoundingMethod', 'Floor','OverflowAction', 'Wrap','ProductMode', 'FullPrecision', 'SumMode', 'FullPrecision')
  data: sig_layer input; max_pooling output; dense_input output
function [max_pooling, dense_input] = max_pooling_layer(sig_layer)

max_pooling = zeros(5,28*28, "single");
max_layer = zeros(5,14*14, "single");
dense_input = zeros(1,980, "single");

% MAX Pooling (max_pooling, max_layer)
for filter_dim=uint32(1:5)
    for i=uint32(1:2:28)
        for j=uint32(1:2:28)
            matrix = [sig_layer(filter_dim, (i-1)*28+j), sig_layer(filter_dim, (i-1)*28+j+1), sig_layer(filter_dim, (i)*28+j), sig_layer(filter_dim, (i)*28+j+1)];
            M = max(matrix);
            if (M == matrix(1))
                I = single(1);
            elseif (M == matrix(2))
                I = single(2);
            elseif (M == matrix(3))
                I = single(3);
            else
                I = single(4);
            end
            max_i = uint32(single(i) + ceil(I/2) - 1);
            max_j = uint32(single(j) + 2-mod(I,2) - 1);
            max_pooling(filter_dim, (max_i-1)*28+max_j) = 1;
            max_layer(filter_dim, ((i+1)/2-1)*14+(j+1)/2) = M;
        end
    end
end
for i=uint32(1:5)
    dense_input((i-1)*14*14 + 1 : (i-1)*14*14 + 14*14) = reshape(max_layer(i,:), [1 14*14]);
end

% pooling = zeros(5,28,28, "single");
% max_layer = zeros(5,14,14, "single");
% dense_input = zeros(1,980, "single");
% 
% % MAX Pooling (max_pooling, max_layer)
% for filter_dim=1:5
%     for i=1:2:28
%         for j=1:2:28
%             matrix = sig_layer(filter_dim,i:i+1,j:j+1);
%             [M,I] = max(matrix);
%             [M2,I2] = max(M);
%             I = [I(I2) I2];
%             max_pooling(filter_dim, I(1), I(2)) = 1;
%             max_layer(filter_dim, (i+1)/2, (j+1)/2) = M2;
%         end
%     end
% end
% for i=1:5
%     for j=1:14
%         dense_input((i-1)*14*14 + (j-1)*14 + 1 : (i-1)*14*14 + (j-1)*14 + 14) = reshape(max_layer(i,j,:), [1 14]);
%     end
% end
